simulink model "Assingment3_3K04_Part1"  (R2017b)
settings: Solver=FixedStepAuto  StartTime=0.0  StopTime=2  FixedStep=1e-3  RelTol=1e-3
undefined symbols (not defined in the file): A0, A1, D0, D1, D10, D11, D12, D13, D2, D3, D4, D5, D6, D7, D8, D9, PTA0, PTA1, PTA2, PTB2, PTB23, PTB3, PTB9, PTC16, PTC17, PTC2, PTC3, PTC4, PTD0, PTD1, PTD2, PTD3
libraries: frdmk64flib x25
settings Model: ExtModeTrigDuration=5  Creator=gagiche  LastModifiedBy=gagiche
settings DataIOCC: LimitDataPoints=on  SaveFormat=Array
settings OptimizationCC: PassReuseOutputArgsAs=Individual arguments  MaxStackSize=64
settings DebuggingCC: UnderspecifiedInitializationDetection=Classic  MergeDetectMultiDrivingBlocksExec=none  SolverPrmCheckMsg=warning  ParameterTunabilityLossMsg=error  StateNameClashWarn=warning  SFUnexpectedBacktrackingDiag=warning  SFNoUnconditionalDefaultTransitionDiag=warning  SFExecutionAtInitializationDiag=none
settings HardwareCC: ProdBitPerPointer=32  ProdBitPerSizeT=32  ProdBitPerPtrDiffT=32  ProdLargestAtomicInteger=Long  ProdLargestAtomicFloat=Double  ProdWordSize=32  ProdHWDeviceType=ARM Compatible->ARM Cortex
settings ModelReferenceCC: PropagateSignalLabelsOutOfModel=off
settings SFSimCC: MATLABDynamicMemAlloc=off
settings RTWCC: SystemTargetFile=ert.tlc  HardwareBoard=NXP FRDM-K64F  TemplateMakefile=ert_default_tmf  GenerateReport=on  Toolchain=GNU Tools for ARM Embedded Processors  IncludeHyperlinkInReport=on  LaunchReport=on  GenerateTraceInfo=on  GenerateTraceReport=on  GenerateTraceReportSl=on  GenerateTraceReportSf=on  GenerateTraceReportEml=on
settings CodeAppCC: ForceParamTrailComments=on  IgnoreCustomStorageClasses=off  OperatorAnnotations=on  SimulinkDataObjDesc=on  SFDataObjDesc=on  InsertBlockDesc=on
settings ConfigComp: CovMetricSettings=dw  CovHtmlReporting=on  CovSaveCumulativeToWorkspaceVar=on  CovSaveSingleToWorkspaceVar=on  CovExternalEMLEnable=off
settings SimscapeCC: SimscapeNormalizeSystem=off

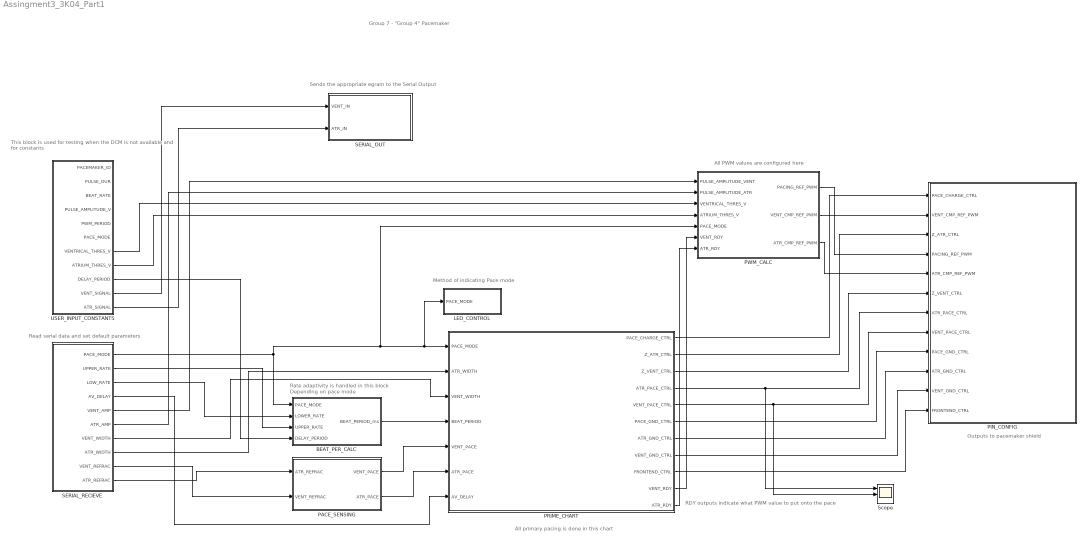
== system Assingment3_3K04_Part1 ==
  note: Group 7 - "Group 4" Pacemaker
  note: RDY outputs indicate what PWM value to put onto the pace
  note: Outputs to pacemaker shield
  note: All primary pacing is done in this chart
  note: Method of indicating Pace mode
  note: Rate adaptivity is handled in this block
      | Depending on pace mode
  note: Sends the appropriate egram to the Serial Output
  note: This block is used for testing when the DCM is not available
      | and for constants
  note: All PWM values are configured here
  note: Read serial data and set default parameters
  BEAT_PER_CALC : Subsystem
  LED_CONTROL : Subsystem
  PACE_SENSING : Subsystem
  "PIN_CONFIG " : Subsystem
  PRIME_CHART : Stateflow chart  TreatAsAtomicUnit=on
  PWM_CALC : Subsystem
  SERIAL_OUT : Subsystem
  SERIAL_RECIEVE : Subsystem
  Scope : Scope  NumInputPorts=3
  USER_INPUT_CONSTANTS : Subsystem
  wires:
  PRIME_CHART/1(PACE_CHARGE_CTRL) -> "PIN_CONFIG "/1(PACE_CHARGE_CTRL)
  PRIME_CHART/2(Z_ATR_CTRL) -> "PIN_CONFIG "/3(Z_ATR_CTRL)
  PRIME_CHART/4(ATR_PACE_CTRL) -> "PIN_CONFIG "/7(ATR_PACE_CTRL), Scope/1
  PRIME_CHART/3(Z_VENT_CTRL) -> "PIN_CONFIG "/6(Z_VENT_CTRL)
  PRIME_CHART/5(VENT_PACE_CTRL) -> Scope/2, "PIN_CONFIG "/8(VENT_PACE_CTRL)
  PRIME_CHART/6(PACE_GND_CTRL) -> "PIN_CONFIG "/9(PACE_GND_CTRL)
  PRIME_CHART/7(ATR_GND_CTRL) -> "PIN_CONFIG "/10(ATR_GND_CTRL)
  PRIME_CHART/8(VENT_GND_CTRL) -> "PIN_CONFIG "/11(VENT_GND_CTRL)
  PRIME_CHART/9(FRONTEND_CTRL) -> "PIN_CONFIG "/12(FRONTEND_CTRL)
  PACE_SENSING/1(VENT_PACE) -> PRIME_CHART/5(VENT_PACE)
  PACE_SENSING/2(ATR_PACE) -> PRIME_CHART/6(ATR_PACE)
  PWM_CALC/2(VENT_CMP_REF_PWM) -> "PIN_CONFIG "/2(VENT_CMP_REF_PWM)
  PWM_CALC/3(ATR_CMP_REF_PWM) -> "PIN_CONFIG "/5(ATR_CMP_REF_PWM)
  PWM_CALC/1(PACING_REF_PWM) -> "PIN_CONFIG "/4(PACING_REF_PWM)
  USER_INPUT_CONSTANTS/7(VENTRICAL_THRES_V) -> PWM_CALC/3(VENTRICAL_THRES_V)
  USER_INPUT_CONSTANTS/8(ATRIUM_THRES_V) -> PWM_CALC/4(ATRIUM_THRES_V)
  SERIAL_RECIEVE/1(PACE_MODE) -> PWM_CALC/5(PACE_MODE), LED_CONTROL/1(PACE_MODE), PRIME_CHART/1(PACE_MODE), BEAT_PER_CALC/1(PACE_MODE)
  SERIAL_RECIEVE/7(VENT_WIDTH) -> PRIME_CHART/3(VENT_WIDTH)
  SERIAL_RECIEVE/3(LOW_RATE) -> BEAT_PER_CALC/2(LOWER_RATE)
  SERIAL_RECIEVE/5(VENT_AMP) -> PWM_CALC/1("PULSE_AMPLITUDE_VENT ")
  SERIAL_RECIEVE/8(ATR_WIDTH) -> PRIME_CHART/2(ATR_WIDTH)
  SERIAL_RECIEVE/9(VENT_REFRAC) -> PACE_SENSING/2(VENT_REFRAC)
  SERIAL_RECIEVE/10(ATR_REFRAC) -> PACE_SENSING/1(ATR_REFRAC)
  SERIAL_RECIEVE/2(UPPER_RATE) -> BEAT_PER_CALC/3(UPPER_RATE)
  SERIAL_RECIEVE/6(ATR_AMP) -> PWM_CALC/2(PULSE_AMPLITUDE_ATR)
  BEAT_PER_CALC/1(BEAT_PERIOD_ms) -> PRIME_CHART/4(BEAT_PERIOD)
  USER_INPUT_CONSTANTS/9(DELAY_PERIOD) -> BEAT_PER_CALC/4(DELAY_PERIOD)
  SERIAL_RECIEVE/4(AV_DELAY) -> PRIME_CHART/7(AV_DELAY)
  PRIME_CHART/10(VENT_RDY) -> PWM_CALC/6(VENT_RDY)
  PRIME_CHART/11(ATR_RDY) -> PWM_CALC/7(ATR_RDY)
  USER_INPUT_CONSTANTS/10(VENT_SIGNAL) -> SERIAL_OUT/1(VENT_IN)
  USER_INPUT_CONSTANTS/11(ATR_SIGNAL) -> SERIAL_OUT/2(ATR_IN)

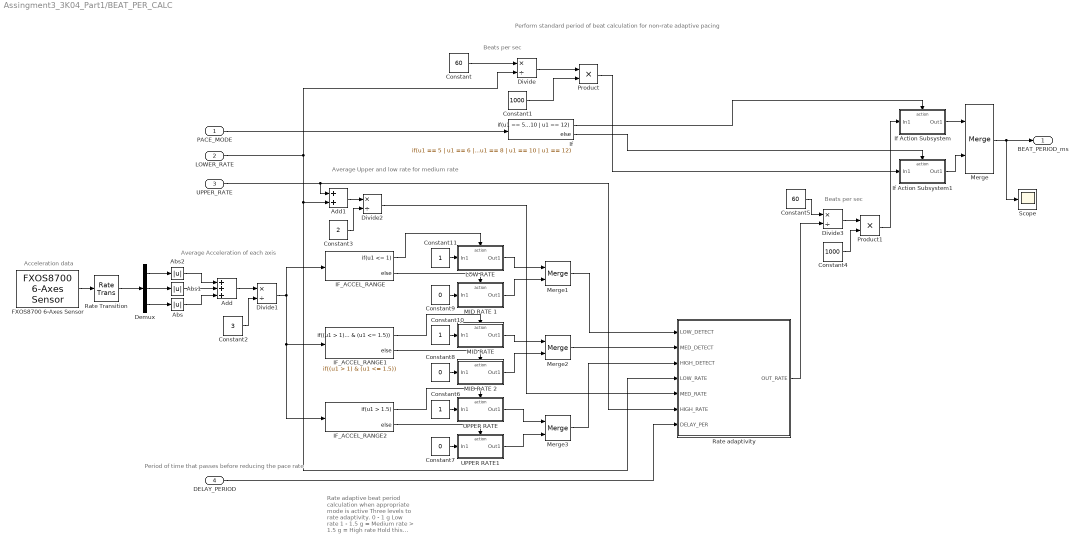
== system Assingment3_3K04_Part1/BEAT_PER_CALC ==
  note: Period of time that passes before reducing the pace rate
  note: Average Upper and low rate for medium rate
  note: Average Acceleration of each axis
  note: Acceleration data
  note: Rate adaptive beat period calculation when appropriate mode is active
      | Three levels to rate adaptivity.
      | 0 - 1 g Low rate
      | 1 - 1.5 g = Medium rate
      | > 1.5 g = High rate
      |
      | Hold this rate for delay_period mseconds
  note: Perform standard period of beat calculation for non-rate adaptive pacing
  note: Beats per sec
  note: Beats per sec
  PACE_MODE : Inport
  LOWER_RATE : Inport  Port=2
  UPPER_RATE : Inport  Port=3
  DELAY_PERIOD : Inport  Port=4
  Abs : Abs  RndMeth=Nearest
  Abs1 : Abs  RndMeth=Nearest
  Abs2 : Abs  RndMeth=Nearest
  Add : Sum  Inputs=3
  Add1 : Sum
  Constant : Constant  Value=60  OutDataTypeStr=double
  Constant1 : Constant  Value=1000  OutDataTypeStr=uint32
  Constant10 : Constant  OutDataTypeStr=double
  Constant11 : Constant  OutDataTypeStr=double
  Constant2 : Constant  Value=3  OutDataTypeStr=double
  Constant3 : Constant  Value=2  OutDataTypeStr=uint8
  Constant4 : Constant  Value=1000  OutDataTypeStr=uint32
  Constant5 : Constant  Value=60  OutDataTypeStr=double
  Constant6 : Constant  OutDataTypeStr=double
  Constant7 : Constant  Value=0  OutDataTypeStr=double
  Constant8 : Constant  Value=0  OutDataTypeStr=double
  Constant9 : Constant  Value=0  OutDataTypeStr=double
  Demux : Demux  Outputs=3
  Divide : Product  Inputs=*/  OutDataTypeStr=double
  Divide1 : Product  Inputs=*/
  Divide2 : Product  Inputs=*/  OutDataTypeStr=uint8
  Divide3 : Product  Inputs=*/  OutDataTypeStr=double
  FXOS8700 6-Axes Sensor : frdmk64flib/FXOS8700 6-Axes Sensor  Activesensor=Accelerometer only  ODR=12.5Hz  HybridODR=400Hz  Accelfullrange=-4g to +4g  SampleTime=0.1
      settings: SourceProductName=Simulink Coder Support Package for NXP FRDM-K64F Board
  IF_ACCEL_RANGE : If  IfExpression=u1 <= 1
  IF_ACCEL_RANGE1 : If  IfExpression=(u1 > 1) & (u1 <= 1.5)
  IF_ACCEL_RANGE2 : If  IfExpression=u1 > 1.5
  If : If  IfExpression=u1 == 5 | u1 == 6 | u1 == 7 | u1 == 8 | u1 == 10 | u1 == 12
  If Action Subsystem : Subsystem  TreatAsAtomicUnit=on
  If Action Subsystem1 : Subsystem  TreatAsAtomicUnit=on
  LOW RATE : Subsystem  TreatAsAtomicUnit=on
  MID RATE : Subsystem  TreatAsAtomicUnit=on
  MID RATE 1 : Subsystem  TreatAsAtomicUnit=on
  MID RATE 2 : Subsystem  TreatAsAtomicUnit=on
  Merge{,1..3} (4 alike) : Merge
  Product : Product  OutDataTypeStr=double
  Product1 : Product  OutDataTypeStr=double
  Rate Transition : RateTransition  OutPortSampleTime=0.001
  Rate adaptivity : Stateflow chart  TreatAsAtomicUnit=on
  Scope : Scope
  UPPER RATE : Subsystem  TreatAsAtomicUnit=on
  UPPER RATE1 : Subsystem  TreatAsAtomicUnit=on
  BEAT_PERIOD_ms : Outport  OutDataTypeStr=double
  wires:
  Divide/1 -> Product/1
  Constant1/1 -> Product/2
  LOWER_RATE/1 -> Rate adaptivity/4(LOW_RATE), Add1/2, Divide/2
  Constant/1 -> Divide/1
  If Action Subsystem/1(Out1) -> Merge/1
  If Action Subsystem1/1(Out1) -> Merge/2
  Merge/1 -> Scope/1, BEAT_PERIOD_ms/1
  PACE_MODE/1 -> If/1
  Demux/2 -> Abs1/1
  Demux/3 -> Abs/1
  Constant2/1 -> Divide1/2
  Demux/1 -> Abs2/1
  Abs2/1 -> Add/1
  Abs1/1 -> Add/2
  Abs/1 -> Add/3
  Add/1 -> Divide1/1
  Divide1/1 -> IF_ACCEL_RANGE2/1, IF_ACCEL_RANGE1/1, IF_ACCEL_RANGE/1
  Product/1 -> If Action Subsystem1/1(In1)
  If/2 -> If Action Subsystem1/Action
  If/1 -> If Action Subsystem/Action
  UPPER_RATE/1 -> Rate adaptivity/6(HIGH_RATE), Add1/1
  Constant3/1 -> Divide2/2
  Add1/1 -> Divide2/1
  Divide3/1 -> Product1/1
  Constant4/1 -> Product1/2
  Constant5/1 -> Divide3/1
  Product1/1 -> If Action Subsystem/1(In1)
  Divide2/1 -> Rate adaptivity/5(MED_RATE)
  IF_ACCEL_RANGE2/1 -> UPPER RATE/Action
  IF_ACCEL_RANGE2/2 -> UPPER RATE1/Action
  Constant6/1 -> UPPER RATE/1(In1)
  Constant7/1 -> UPPER RATE1/1(In1)
  IF_ACCEL_RANGE1/1 -> MID RATE/Action
  Constant8/1 -> MID RATE 2/1(In1)
  IF_ACCEL_RANGE1/2 -> MID RATE 2/Action
  IF_ACCEL_RANGE/1 -> LOW RATE/Action
  IF_ACCEL_RANGE/2 -> MID RATE 1/Action
  Constant9/1 -> MID RATE 1/1(In1)
  Constant10/1 -> MID RATE/1(In1)
  Constant11/1 -> LOW RATE/1(In1)
  LOW RATE/1(Out1) -> Merge1/1
  MID RATE 1/1(Out1) -> Merge1/2
  Merge1/1 -> Rate adaptivity/1(LOW_DETECT)
  Merge2/1 -> Rate adaptivity/2(MED_DETECT)
  MID RATE/1(Out1) -> Merge2/1
  MID RATE 2/1(Out1) -> Merge2/2
  UPPER RATE/1(Out1) -> Merge3/1
  UPPER RATE1/1(Out1) -> Merge3/2
  Merge3/1 -> Rate adaptivity/3(HIGH_DETECT)
  DELAY_PERIOD/1 -> Rate adaptivity/7(DELAY_PER)
  Rate adaptivity/1(OUT_RATE) -> Divide3/2
  FXOS8700 6-Axes Sensor/1 -> Rate Transition/1
  Rate Transition/1 -> Demux/1

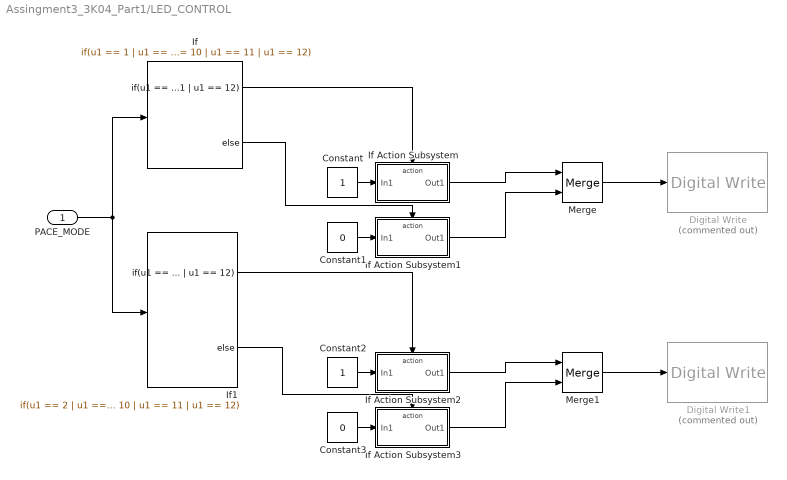
== system Assingment3_3K04_Part1/LED_CONTROL ==
  PACE_MODE : Inport
  Constant : Constant  OutDataTypeStr=boolean
  Constant1 : Constant  Value=0  OutDataTypeStr=boolean
  Constant2 : Constant  OutDataTypeStr=boolean
  Constant3 : Constant  Value=0  OutDataTypeStr=boolean
  Digital Write : frdmk64flib/Digital Write  Commented=on  Whichpin=GREEN_LED
      settings: SourceProductName=Simulink Coder Support Package for NXP FRDM-K64F Board
  Digital Write1 : frdmk64flib/Digital Write  Commented=on  Whichpin=RED_LED
      settings: SourceProductName=Simulink Coder Support Package for NXP FRDM-K64F Board
  If : If  IfExpression=u1 == 1 | u1 == 3 | u1 == 5 | u1 == 7 | u1 == 9 | u1 == 10 | u1 == 11 | u1 == 12
  If Action Subsystem : Subsystem  TreatAsAtomicUnit=on
  If Action Subsystem1 : Subsystem  TreatAsAtomicUnit=on
  If Action Subsystem2 : Subsystem  TreatAsAtomicUnit=on
  If Action Subsystem3 : Subsystem  TreatAsAtomicUnit=on
  If1 : If  IfExpression=u1 == 2 | u1 == 4 | u1 == 6 | u1 == 8 | u1 == 9 | u1 == 10 | u1 == 11 | u1 == 12
  Merge : Merge
  Merge1 : Merge
  wires:
  PACE_MODE/1 -> If1/1, If/1
  If/1 -> If Action Subsystem/Action
  If/2 -> If Action Subsystem1/Action
  Constant/1 -> If Action Subsystem/1(In1)
  Constant1/1 -> If Action Subsystem1/1(In1)
  Merge/1 -> Digital Write/1
  If Action Subsystem/1(Out1) -> Merge/1
  If Action Subsystem1/1(Out1) -> Merge/2
  Constant3/1 -> If Action Subsystem3/1(In1)
  If Action Subsystem3/1(Out1) -> Merge1/2
  If Action Subsystem2/1(Out1) -> Merge1/1
  Constant2/1 -> If Action Subsystem2/1(In1)
  Merge1/1 -> Digital Write1/1
  If1/2 -> If Action Subsystem3/Action
  If1/1 -> If Action Subsystem2/Action

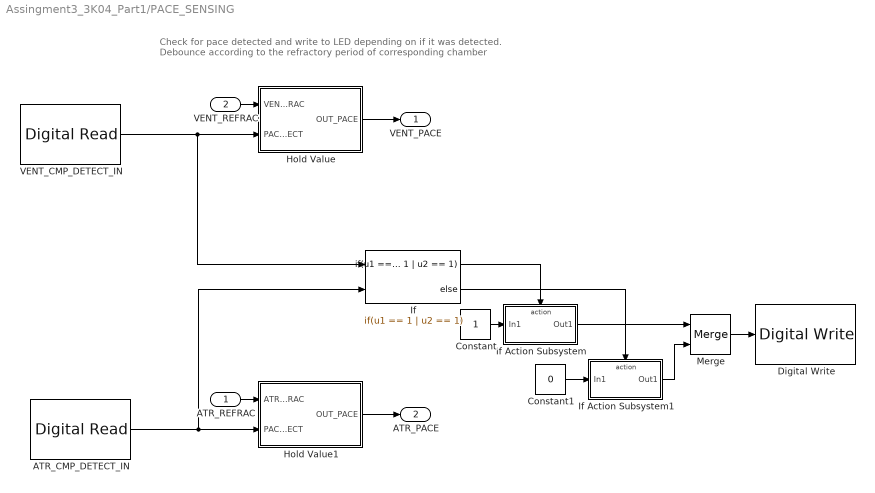
== system Assingment3_3K04_Part1/PACE_SENSING ==
  note: Check for pace detected and write to LED depending on if it was detected.
      | Debounce according to the refractory period of corresponding chamber
  ATR_REFRAC : Inport
  VENT_REFRAC : Inport  Port=2
  ATR_CMP_DETECT_IN : frdmk64flib/Digital Read  Whichpin=PTC16 (D0)  SampleTime=-1
      settings: SourceProductName=Simulink Coder Support Package for NXP FRDM-K64F Board
  Constant : Constant
  Constant1 : Constant  Value=0
  Digital Write : frdmk64flib/Digital Write  Whichpin=GREEN_LED
      settings: SourceProductName=Simulink Coder Support Package for NXP FRDM-K64F Board
  Hold Value : Stateflow chart  TreatAsAtomicUnit=on
  Hold Value1 : Stateflow chart  TreatAsAtomicUnit=on
  If : If  NumInputs=2  IfExpression=u1 == 1 | u2 == 1
  If Action Subsystem : Subsystem  TreatAsAtomicUnit=on
  If Action Subsystem1 : Subsystem  TreatAsAtomicUnit=on
  Merge : Merge
  VENT_CMP_DETECT_IN : frdmk64flib/Digital Read  Whichpin=PTC17 (D1)  SampleTime=-1
      settings: SourceProductName=Simulink Coder Support Package for NXP FRDM-K64F Board
  VENT_PACE : Outport  OutDataTypeStr=boolean
  ATR_PACE : Outport  Port=2  OutDataTypeStr=boolean
  wires:
  VENT_CMP_DETECT_IN/1 -> Hold Value/2(PACE_DETECT), If/1
  Merge/1 -> Digital Write/1
  If/1 -> If Action Subsystem/Action
  Constant/1 -> If Action Subsystem/1(In1)
  Constant1/1 -> If Action Subsystem1/1(In1)
  If/2 -> If Action Subsystem1/Action
  If Action Subsystem1/1(Out1) -> Merge/2
  If Action Subsystem/1(Out1) -> Merge/1
  ATR_CMP_DETECT_IN/1 -> If/2, Hold Value1/2(PACE_DETECT)
  VENT_REFRAC/1 -> Hold Value/1(VENT_REFRAC)
  Hold Value/1(OUT_PACE) -> VENT_PACE/1
  ATR_REFRAC/1 -> Hold Value1/1(ATR_REFRAC)
  Hold Value1/1(OUT_PACE) -> ATR_PACE/1

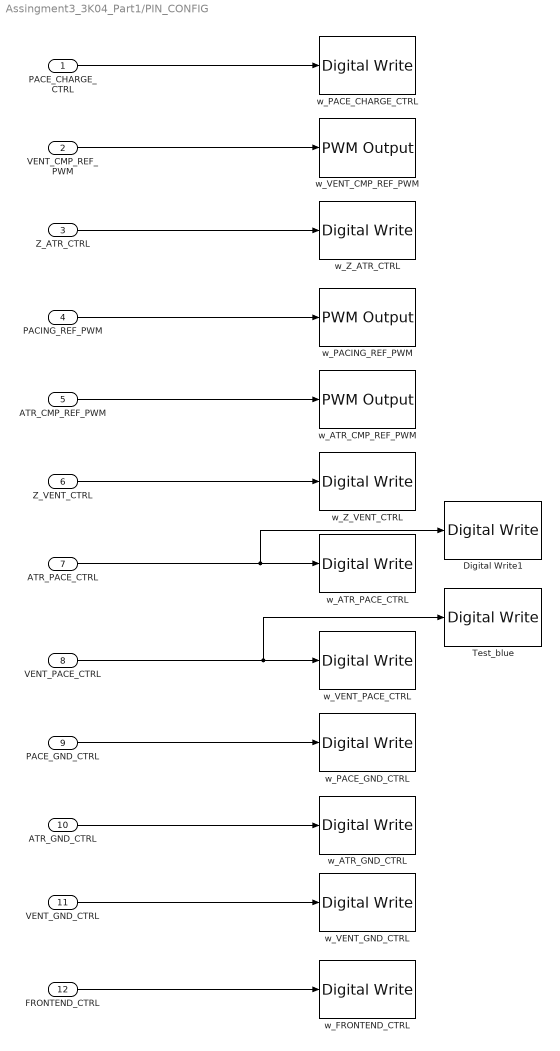
== system Assingment3_3K04_Part1/PIN_CONFIG  ==
  PACE_CHARGE_CTRL : Inport
  VENT_CMP_REF_PWM : Inport  Port=2
  Z_ATR_CTRL : Inport  Port=3
  PACING_REF_PWM : Inport  Port=4
  ATR_CMP_REF_PWM : Inport  Port=5
  Z_VENT_CTRL : Inport  Port=6
  ATR_PACE_CTRL : Inport  Port=7
  VENT_PACE_CTRL : Inport  Port=8
  PACE_GND_CTRL : Inport  Port=9
  ATR_GND_CTRL : Inport  Port=10
  VENT_GND_CTRL : Inport  Port=11
  FRONTEND_CTRL : Inport  Port=12
  Digital Write1 : frdmk64flib/Digital Write  Whichpin=RED_LED
      settings: SourceProductName=Simulink Coder Support Package for NXP FRDM-K64F Board
  Test_blue : frdmk64flib/Digital Write  Whichpin=BLUE_LED
      settings: SourceProductName=Simulink Coder Support Package for NXP FRDM-K64F Board
  w_ATR_CMP_REF_PWM : frdmk64flib/PWM Output  Whichpin=PTC2 (D6)  InitialFrequency=1000  InitialDutyCycle=0
      settings: SourceProductName=Simulink Coder Support Package for NXP FRDM-K64F Board
  w_ATR_GND_CTRL : frdmk64flib/Digital Write  Whichpin=PTD2 (D11)
      settings: SourceProductName=Simulink Coder Support Package for NXP FRDM-K64F Board
  w_ATR_PACE_CTRL : frdmk64flib/Digital Write  Whichpin=PTA0 (D8)
      settings: SourceProductName=Simulink Coder Support Package for NXP FRDM-K64F Board
  w_FRONTEND_CTRL : frdmk64flib/Digital Write  Whichpin=PTD1 (D13)
      settings: SourceProductName=Simulink Coder Support Package for NXP FRDM-K64F Board
  w_PACE_CHARGE_CTRL : frdmk64flib/Digital Write  Whichpin=PTB9 (D2)
      settings: SourceProductName=Simulink Coder Support Package for NXP FRDM-K64F Board
  w_PACE_GND_CTRL : frdmk64flib/Digital Write  Whichpin=PTD0 (D10)
      settings: SourceProductName=Simulink Coder Support Package for NXP FRDM-K64F Board
  w_PACING_REF_PWM : frdmk64flib/PWM Output  Whichpin=PTA2 (D5)  InitialFrequency=1000  InitialDutyCycle=0
      settings: SourceProductName=Simulink Coder Support Package for NXP FRDM-K64F Board
  w_VENT_CMP_REF_PWM : frdmk64flib/PWM Output  Whichpin=PTA1 (D3)  InitialFrequency=1000  InitialDutyCycle=0
      settings: SourceProductName=Simulink Coder Support Package for NXP FRDM-K64F Board
  w_VENT_GND_CTRL : frdmk64flib/Digital Write  Whichpin=PTD3 (D12)
      settings: SourceProductName=Simulink Coder Support Package for NXP FRDM-K64F Board
  w_VENT_PACE_CTRL : frdmk64flib/Digital Write  Whichpin=PTC4 (D9)
      settings: SourceProductName=Simulink Coder Support Package for NXP FRDM-K64F Board
  w_Z_ATR_CTRL : frdmk64flib/Digital Write  Whichpin=PTB23 (D4)
      settings: SourceProductName=Simulink Coder Support Package for NXP FRDM-K64F Board
  w_Z_VENT_CTRL : frdmk64flib/Digital Write  Whichpin=PTC3 (D7)
      settings: SourceProductName=Simulink Coder Support Package for NXP FRDM-K64F Board
  wires:
  PACE_CHARGE_CTRL/1 -> w_PACE_CHARGE_CTRL/1
  VENT_CMP_REF_PWM/1 -> w_VENT_CMP_REF_PWM/1
  Z_ATR_CTRL/1 -> w_Z_ATR_CTRL/1
  PACING_REF_PWM/1 -> w_PACING_REF_PWM/1
  ATR_CMP_REF_PWM/1 -> w_ATR_CMP_REF_PWM/1
  Z_VENT_CTRL/1 -> w_Z_VENT_CTRL/1
  ATR_PACE_CTRL/1 -> Digital Write1/1, w_ATR_PACE_CTRL/1
  VENT_PACE_CTRL/1 -> Test_blue/1, w_VENT_PACE_CTRL/1
  PACE_GND_CTRL/1 -> w_PACE_GND_CTRL/1
  ATR_GND_CTRL/1 -> w_ATR_GND_CTRL/1
  VENT_GND_CTRL/1 -> w_VENT_GND_CTRL/1
  FRONTEND_CTRL/1 -> w_FRONTEND_CTRL/1

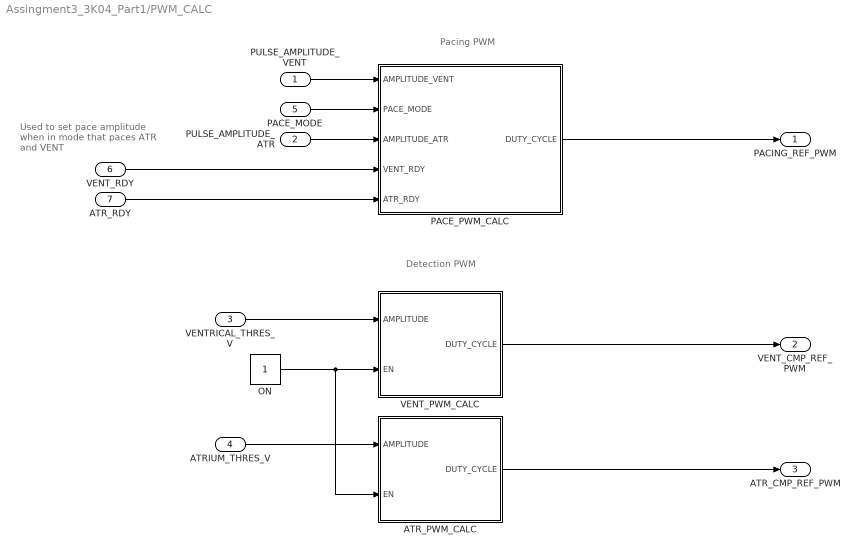
== system Assingment3_3K04_Part1/PWM_CALC ==
  note: Used to set pace amplitude
      | when in mode that paces ATR and VENT
  note: Pacing PWM
  note: Detection PWM
  "PULSE_AMPLITUDE_VENT " : Inport
  PULSE_AMPLITUDE_ATR : Inport  Port=2
  VENTRICAL_THRES_V : Inport  Port=3
  ATRIUM_THRES_V : Inport  Port=4
  PACE_MODE : Inport  Port=5
  VENT_RDY : Inport  Port=6
  ATR_RDY : Inport  Port=7
  ATR_PWM_CALC : Subsystem
  ON : Constant  OutDataTypeStr=boolean
  PACE_PWM_CALC : Subsystem
  VENT_PWM_CALC : Subsystem
  PACING_REF_PWM : Outport
  VENT_CMP_REF_PWM : Outport  Port=2
  ATR_CMP_REF_PWM : Outport  Port=3
  wires:
  ON/1 -> ATR_PWM_CALC/2(EN), VENT_PWM_CALC/2(EN)
  "PULSE_AMPLITUDE_VENT "/1 -> PACE_PWM_CALC/1(AMPLITUDE_VENT)
  VENTRICAL_THRES_V/1 -> VENT_PWM_CALC/1(AMPLITUDE)
  ATRIUM_THRES_V/1 -> ATR_PWM_CALC/1(AMPLITUDE)
  ATR_PWM_CALC/1(DUTY_CYCLE) -> ATR_CMP_REF_PWM/1
  VENT_PWM_CALC/1(DUTY_CYCLE) -> VENT_CMP_REF_PWM/1
  PACE_PWM_CALC/1(DUTY_CYCLE) -> PACING_REF_PWM/1
  PULSE_AMPLITUDE_ATR/1 -> PACE_PWM_CALC/3(AMPLITUDE_ATR)
  PACE_MODE/1 -> PACE_PWM_CALC/2(PACE_MODE)
  VENT_RDY/1 -> PACE_PWM_CALC/4(VENT_RDY)
  ATR_RDY/1 -> PACE_PWM_CALC/5(ATR_RDY)

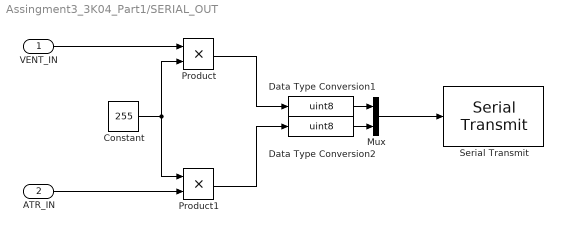
== system Assingment3_3K04_Part1/SERIAL_OUT ==
  VENT_IN : Inport
  ATR_IN : Inport  Port=2
  Constant : Constant  Value=255
  Data Type Conversion1 : DataTypeConversion  OutDataTypeStr=uint8
  Data Type Conversion2 : DataTypeConversion  OutDataTypeStr=uint8
  Mux : Mux  Inputs=2
  Product : Product
  Product1 : Product
  Serial Transmit : frdmk64flib/Serial Transmit  SCIModule=0  Baudrate=uint32(9600)  Parity=None  StopBits=1  HardwareFlowControl=None  ByteOrder=LittleEndian  BlockingMode=on  OutputStatus=off
      settings: SourceProductName=Simulink Coder Support Package for NXP FRDM-K64F Board
  wires:
  Constant/1 -> Product1/1, Product/2
  Product/1 -> Data Type Conversion1/1
  Product1/1 -> Data Type Conversion2/1
  Data Type Conversion1/1 -> Mux/1
  Data Type Conversion2/1 -> Mux/2
  Mux/1 -> Serial Transmit/1
  VENT_IN/1 -> Product/1
  ATR_IN/1 -> Product1/2

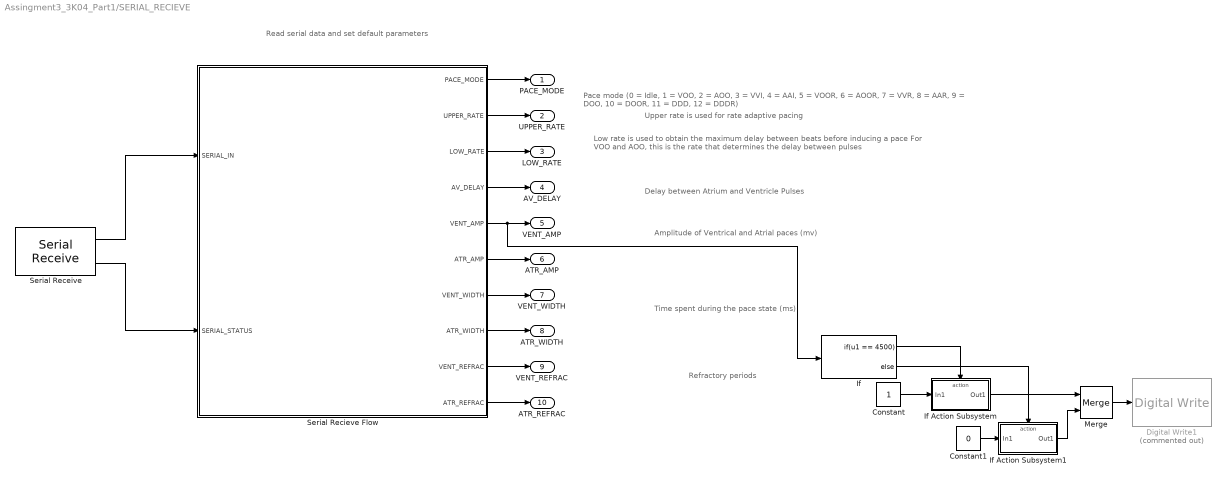
== system Assingment3_3K04_Part1/SERIAL_RECIEVE ==
  note: Read serial data and set default parameters
  note: Pace mode (0 = Idle, 1 = VOO, 2 = AOO, 3 = VVI, 4 = AAI, 5 = VOOR, 6 = AOOR, 7 = VVR, 8 = AAR, 9 = DOO, 10 = DOOR, 11 = DDD, 12 = DDDR)
  note: Amplitude of Ventrical and Atrial paces (mv)
  note: Delay between Atrium and Ventricle Pulses
  note: Refractory periods
  note: Upper rate is used for rate adaptive pacing
  note: Time spent during the pace state (ms)
  note: Low rate is used to obtain the maximum delay between beats before inducing a pace
      | For VOO and AOO, this is the rate that determines the delay between pulses
  Constant : Constant
  Constant1 : Constant  Value=0
  Digital Write1 : frdmk64flib/Digital Write  Commented=on  Whichpin=GREEN_LED
      settings: SourceProductName=Simulink Coder Support Package for NXP FRDM-K64F Board
  If : If  IfExpression=u1 == 4500
  If Action Subsystem : Subsystem  TreatAsAtomicUnit=on
  If Action Subsystem1 : Subsystem  TreatAsAtomicUnit=on
  Merge : Merge
  Serial Receive : frdmk64flib/Serial Receive  SCIModule=0  Baudrate=uint32(9600)  Parity=None  StopBits=1  HardwareFlowControl=None  ByteOrder=LittleEndian  DataType=uint8  DataLength=10  BlockingMode=off  OutputStatus=on  SampleTime=-1
      settings: SourceProductName=Simulink Coder Support Package for NXP FRDM-K64F Board
  Serial Recieve Flow : Stateflow chart  TreatAsAtomicUnit=on
  PACE_MODE : Outport  OutDataTypeStr=uint8
  UPPER_RATE : Outport  Port=2  OutDataTypeStr=uint8
  LOW_RATE : Outport  Port=3  OutDataTypeStr=uint8
  AV_DELAY : Outport  Port=4
  VENT_AMP : Outport  Port=5
  ATR_AMP : Outport  Port=6
  VENT_WIDTH : Outport  Port=7
  ATR_WIDTH : Outport  Port=8
  VENT_REFRAC : Outport  Port=9
  ATR_REFRAC : Outport  Port=10
  wires:
  Serial Recieve Flow/1(PACE_MODE) -> PACE_MODE/1
  Serial Recieve Flow/6(ATR_AMP) -> ATR_AMP/1
  Serial Recieve Flow/7(VENT_WIDTH) -> VENT_WIDTH/1
  Serial Recieve Flow/4(AV_DELAY) -> AV_DELAY/1
  Serial Recieve Flow/2(UPPER_RATE) -> UPPER_RATE/1
  Serial Recieve Flow/9(VENT_REFRAC) -> VENT_REFRAC/1
  Serial Recieve Flow/5(VENT_AMP) -> If/1, VENT_AMP/1
  Serial Recieve Flow/10(ATR_REFRAC) -> ATR_REFRAC/1
  Serial Recieve Flow/8(ATR_WIDTH) -> ATR_WIDTH/1
  Serial Recieve Flow/3(LOW_RATE) -> LOW_RATE/1
  If Action Subsystem1/1(Out1) -> Merge/2
  If/2 -> If Action Subsystem1/Action
  Constant/1 -> If Action Subsystem/1(In1)
  If/1 -> If Action Subsystem/Action
  Merge/1 -> Digital Write1/1
  Constant1/1 -> If Action Subsystem1/1(In1)
  If Action Subsystem/1(Out1) -> Merge/1
  Serial Receive/1 -> Serial Recieve Flow/1(SERIAL_IN)
  Serial Receive/2 -> Serial Recieve Flow/2(SERIAL_STATUS)

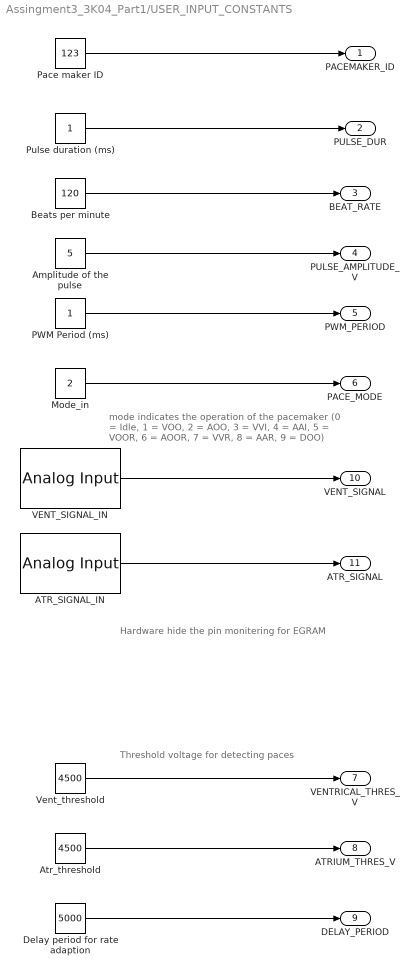
== system Assingment3_3K04_Part1/USER_INPUT_CONSTANTS ==
  note: Hardware hide the pin monitering for EGRAM
  note: Threshold voltage for detecting paces
  note: mode indicates the operation of the pacemaker
      | (0 = Idle, 1 = VOO, 2 = AOO, 3 = VVI, 4 = AAI, 5 = VOOR, 6 = AOOR, 7 = VVR, 8 = AAR, 9 = DOO)
  ATR_SIGNAL_IN : frdmk64flib/Analog Input  Whichpin=PTB2 (A0)  SampleTime=-1
      settings: SourceProductName=Simulink Coder Support Package for NXP FRDM-K64F Board
  Amplitude of the pulse : Constant  Value=5
  Atr_threshold : Constant  Value=4500  OutDataTypeStr=double
  Beats per minute : Constant  Value=120
  Delay period for rate adaption : Constant  Value=5000  OutDataTypeStr=double
  Mode_in : Constant  Value=2  OutDataTypeStr=uint16
  PWM Period (ms) : Constant  OutDataTypeStr=uint16
  Pace maker ID : Constant  Value=123  OutDataTypeStr=double
  Pulse duration (ms) : Constant  OutDataTypeStr=double
  VENT_SIGNAL_IN : frdmk64flib/Analog Input  Whichpin=PTB3 (A1)  SampleTime=-1
      settings: SourceProductName=Simulink Coder Support Package for NXP FRDM-K64F Board
  Vent_threshold : Constant  Value=4500  OutDataTypeStr=double
  PACEMAKER_ID : Outport  OutDataTypeStr=double
  "PULSE_DUR " : Outport  Port=2  OutDataTypeStr=double
  "BEAT_RATE " : Outport  Port=3
  "PULSE_AMPLITUDE_V " : Outport  Port=4
  PWM_PERIOD : Outport  Port=5
  PACE_MODE : Outport  Port=6
  VENTRICAL_THRES_V : Outport  Port=7
  ATRIUM_THRES_V : Outport  Port=8
  DELAY_PERIOD : Outport  Port=9
  VENT_SIGNAL : Outport  Port=10
  ATR_SIGNAL : Outport  Port=11
  wires:
  Pulse duration (ms)/1 -> "PULSE_DUR "/1
  Beats per minute/1 -> "BEAT_RATE "/1
  Amplitude of the pulse/1 -> "PULSE_AMPLITUDE_V "/1
  PWM Period (ms)/1 -> PWM_PERIOD/1
  Mode_in/1 -> PACE_MODE/1
  Vent_threshold/1 -> VENTRICAL_THRES_V/1
  Atr_threshold/1 -> ATRIUM_THRES_V/1
  Pace maker ID/1 -> PACEMAKER_ID/1
  Delay period for rate adaption/1 -> DELAY_PERIOD/1
  VENT_SIGNAL_IN/1 -> VENT_SIGNAL/1
  ATR_SIGNAL_IN/1 -> ATR_SIGNAL/1

== system Assingment3_3K04_Part1/BEAT_PER_CALC/If Action Subsystem ==
  In1 : Inport
  Action Port : ActionPort  ActionType=then
  Out1 : Outport
  wires:
  In1/1 -> Out1/1

== system Assingment3_3K04_Part1/BEAT_PER_CALC/If Action Subsystem1 ==
  In1 : Inport
  Action Port : ActionPort  ActionType=else
  Out1 : Outport
  wires:
  In1/1 -> Out1/1

== system Assingment3_3K04_Part1/BEAT_PER_CALC/LOW RATE ==
  In1 : Inport
  Action Port : ActionPort  ActionType=then
  Out1 : Outport
  wires:
  In1/1 -> Out1/1

== system Assingment3_3K04_Part1/BEAT_PER_CALC/MID RATE ==
  In1 : Inport
  Action Port : ActionPort  ActionType=then
  Out1 : Outport
  wires:
  In1/1 -> Out1/1

== system Assingment3_3K04_Part1/BEAT_PER_CALC/MID RATE 1 ==
  In1 : Inport
  Action Port : ActionPort  ActionType=else
  Out1 : Outport
  wires:
  In1/1 -> Out1/1

== system Assingment3_3K04_Part1/BEAT_PER_CALC/MID RATE 2 ==
  In1 : Inport
  Action Port : ActionPort  ActionType=else
  Out1 : Outport
  wires:
  In1/1 -> Out1/1

== system Assingment3_3K04_Part1/BEAT_PER_CALC/UPPER RATE ==
  In1 : Inport
  Action Port : ActionPort  ActionType=then
  Out1 : Outport
  wires:
  In1/1 -> Out1/1

== system Assingment3_3K04_Part1/BEAT_PER_CALC/UPPER RATE1 ==
  In1 : Inport
  Action Port : ActionPort  ActionType=else
  Out1 : Outport
  wires:
  In1/1 -> Out1/1

== system Assingment3_3K04_Part1/LED_CONTROL/If Action Subsystem ==
  In1 : Inport
  Action Port : ActionPort  ActionType=then
  Out1 : Outport
  wires:
  In1/1 -> Out1/1

== system Assingment3_3K04_Part1/LED_CONTROL/If Action Subsystem1 ==
  In1 : Inport
  Action Port : ActionPort  ActionType=else
  Out1 : Outport
  wires:
  In1/1 -> Out1/1

== system Assingment3_3K04_Part1/LED_CONTROL/If Action Subsystem2 ==
  In1 : Inport
  Action Port : ActionPort  ActionType=then
  Out1 : Outport
  wires:
  In1/1 -> Out1/1

== system Assingment3_3K04_Part1/LED_CONTROL/If Action Subsystem3 ==
  In1 : Inport
  Action Port : ActionPort  ActionType=else
  Out1 : Outport
  wires:
  In1/1 -> Out1/1

== system Assingment3_3K04_Part1/PACE_SENSING/If Action Subsystem ==
  In1 : Inport
  Action Port : ActionPort  ActionType=then
  Out1 : Outport
  wires:
  In1/1 -> Out1/1

== system Assingment3_3K04_Part1/PACE_SENSING/If Action Subsystem1 ==
  In1 : Inport
  Action Port : ActionPort  ActionType=else
  Out1 : Outport
  wires:
  In1/1 -> Out1/1

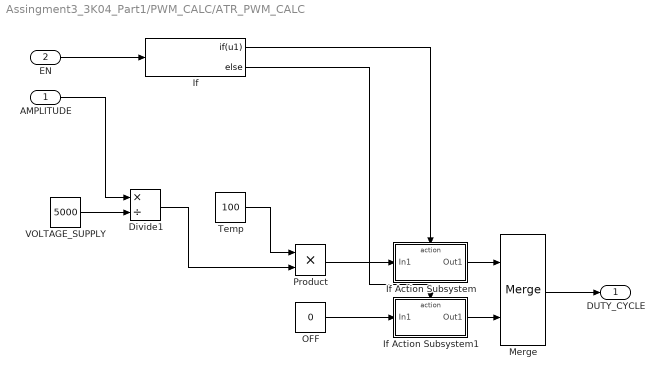
== system Assingment3_3K04_Part1/PWM_CALC/ATR_PWM_CALC ==
  AMPLITUDE : Inport  OutDataTypeStr=double
  EN : Inport  Port=2  OutDataTypeStr=boolean
  Divide1 : Product  Inputs=*/  OutDataTypeStr=double
  If : If  IfExpression=u1
  If Action Subsystem : Subsystem  TreatAsAtomicUnit=on
  If Action Subsystem1 : Subsystem  TreatAsAtomicUnit=on
  Merge : Merge
  OFF : Constant  Value=0  OutDataTypeStr=uint32
  Product : Product  OutDataTypeStr=uint32
  "Temp " : Constant  Value=100  OutDataTypeStr=double
  "VOLTAGE_SUPPLY " : Constant  Value=5000  OutDataTypeStr=double
  DUTY_CYCLE : Outport  OutDataTypeStr=uint32  LockScale=on
  wires:
  "VOLTAGE_SUPPLY "/1 -> Divide1/2
  "Temp "/1 -> Product/1
  EN/1 -> If/1
  Merge/1 -> DUTY_CYCLE/1
  If Action Subsystem/1(Out1) -> Merge/1
  If Action Subsystem1/1(Out1) -> Merge/2
  Product/1 -> If Action Subsystem/1(In1)
  If/1 -> If Action Subsystem/Action
  If/2 -> If Action Subsystem1/Action
  OFF/1 -> If Action Subsystem1/1(In1)
  AMPLITUDE/1 -> Divide1/1
  Divide1/1 -> Product/2

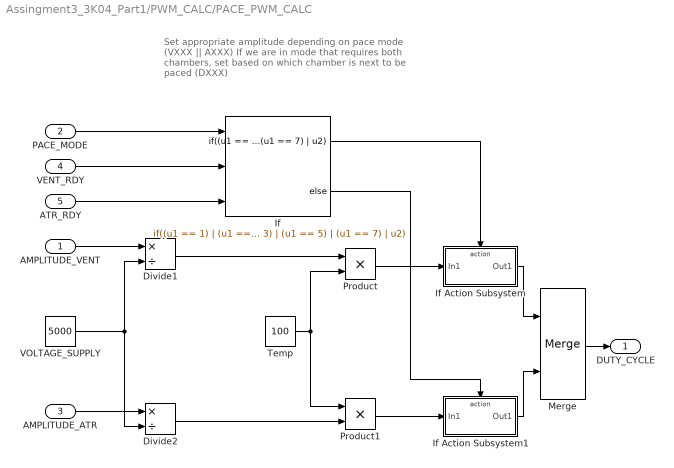
== system Assingment3_3K04_Part1/PWM_CALC/PACE_PWM_CALC ==
  note: Set appropriate amplitude depending on pace mode
      | (VXXX || AXXX)
      | If we are in mode that requires both chambers, set
      | based on which chamber is next to be paced
      | (DXXX)
  AMPLITUDE_VENT : Inport
  PACE_MODE : Inport  Port=2  OutDataTypeStr=uint8
  AMPLITUDE_ATR : Inport  Port=3  OutDataTypeStr=double
  VENT_RDY : Inport  Port=4
  ATR_RDY : Inport  Port=5
  Divide1 : Product  Inputs=*/  OutDataTypeStr=double
  Divide2 : Product  Inputs=*/  OutDataTypeStr=double
  If : If  NumInputs=3  IfExpression=(u1 == 1) | (u1 == 3) | (u1 == 5) | (u1 == 7) | u2
  If Action Subsystem : Subsystem  TreatAsAtomicUnit=on
  If Action Subsystem1 : Subsystem  TreatAsAtomicUnit=on
  Merge : Merge
  Product : Product  OutDataTypeStr=uint32
  Product1 : Product  OutDataTypeStr=uint32
  "Temp " : Constant  Value=100  OutDataTypeStr=double
  "VOLTAGE_SUPPLY " : Constant  Value=5000  OutDataTypeStr=double
  DUTY_CYCLE : Outport  OutDataTypeStr=uint32  LockScale=on
  wires:
  "VOLTAGE_SUPPLY "/1 -> Divide1/2, Divide2/2
  "Temp "/1 -> Product1/1, Product/2
  PACE_MODE/1 -> If/1
  If Action Subsystem/1(Out1) -> Merge/1
  If Action Subsystem1/1(Out1) -> Merge/2
  Product/1 -> If Action Subsystem/1(In1)
  If/1 -> If Action Subsystem/Action
  If/2 -> If Action Subsystem1/Action
  AMPLITUDE_VENT/1 -> Divide1/1
  Divide2/1 -> Product1/2
  AMPLITUDE_ATR/1 -> Divide2/1
  Product1/1 -> If Action Subsystem1/1(In1)
  Divide1/1 -> Product/1
  Merge/1 -> DUTY_CYCLE/1
  VENT_RDY/1 -> If/2
  ATR_RDY/1 -> If/3

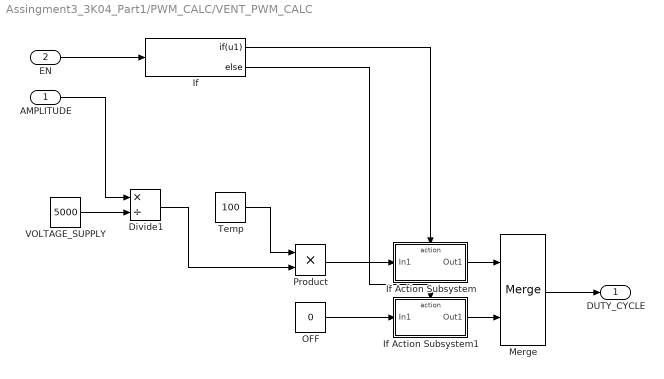
== system Assingment3_3K04_Part1/PWM_CALC/VENT_PWM_CALC ==
  AMPLITUDE : Inport  OutDataTypeStr=double
  EN : Inport  Port=2  OutDataTypeStr=boolean
  Divide1 : Product  Inputs=*/  OutDataTypeStr=double
  If : If  IfExpression=u1
  If Action Subsystem : Subsystem  TreatAsAtomicUnit=on
  If Action Subsystem1 : Subsystem  TreatAsAtomicUnit=on
  Merge : Merge
  OFF : Constant  Value=0  OutDataTypeStr=uint32
  Product : Product  OutDataTypeStr=uint32
  "Temp " : Constant  Value=100  OutDataTypeStr=double
  "VOLTAGE_SUPPLY " : Constant  Value=5000  OutDataTypeStr=double
  DUTY_CYCLE : Outport  OutDataTypeStr=uint32  LockScale=on
  wires:
  "VOLTAGE_SUPPLY "/1 -> Divide1/2
  "Temp "/1 -> Product/1
  EN/1 -> If/1
  Merge/1 -> DUTY_CYCLE/1
  If Action Subsystem/1(Out1) -> Merge/1
  If Action Subsystem1/1(Out1) -> Merge/2
  Product/1 -> If Action Subsystem/1(In1)
  If/1 -> If Action Subsystem/Action
  If/2 -> If Action Subsystem1/Action
  OFF/1 -> If Action Subsystem1/1(In1)
  AMPLITUDE/1 -> Divide1/1
  Divide1/1 -> Product/2

== system Assingment3_3K04_Part1/SERIAL_RECIEVE/If Action Subsystem ==
  In1 : Inport
  Action Port : ActionPort  ActionType=then
  Out1 : Outport
  wires:
  In1/1 -> Out1/1

== system Assingment3_3K04_Part1/SERIAL_RECIEVE/If Action Subsystem1 ==
  In1 : Inport
  Action Port : ActionPort  ActionType=else
  Out1 : Outport
  wires:
  In1/1 -> Out1/1

== system Assingment3_3K04_Part1/PWM_CALC/ATR_PWM_CALC/If Action Subsystem ==
  In1 : Inport
  Action Port : ActionPort  ActionType=then
  Out1 : Outport
  wires:
  In1/1 -> Out1/1

== system Assingment3_3K04_Part1/PWM_CALC/ATR_PWM_CALC/If Action Subsystem1 ==
  In1 : Inport
  Action Port : ActionPort  ActionType=else
  Out1 : Outport
  wires:
  In1/1 -> Out1/1

== system Assingment3_3K04_Part1/PWM_CALC/PACE_PWM_CALC/If Action Subsystem ==
  In1 : Inport
  Action Port : ActionPort  ActionType=then
  Out1 : Outport
  wires:
  In1/1 -> Out1/1

== system Assingment3_3K04_Part1/PWM_CALC/PACE_PWM_CALC/If Action Subsystem1 ==
  In1 : Inport
  Action Port : ActionPort  ActionType=else
  Out1 : Outport
  wires:
  In1/1 -> Out1/1

== system Assingment3_3K04_Part1/PWM_CALC/VENT_PWM_CALC/If Action Subsystem ==
  In1 : Inport
  Action Port : ActionPort  ActionType=then
  Out1 : Outport
  wires:
  In1/1 -> Out1/1

== system Assingment3_3K04_Part1/PWM_CALC/VENT_PWM_CALC/If Action Subsystem1 ==
  In1 : Inport
  Action Port : ActionPort  ActionType=else
  Out1 : Outport
  wires:
  In1/1 -> Out1/1

== stateflow chart Assingment3_3K04_Part1/BEAT_PER_CALC/Rate adaptivity ==
  settings: sampleTime=0.001
  note: Based on the detected acceleration, jump to the appropriate rate response
  state LOW_RATE
    entry:
    OUT_RATE = LOW_RATE;
  state MED_RATE
    entry:
    OUT_RATE = MED_RATE;
  note: Reduce the rate after a period of no accerlation corresponding to the rate
  state HIGH_RATE
    entry:
    OUT_RATE = HIGH_RATE;
  (default) -> LOW_RATE
  LOW_RATE -> LOW_RATE [order 3] : [after(200,msec)]
  MED_RATE -> LOW_RATE [order 2] : [after(DELAY_PER, msec)]
  LOW_RATE -> HIGH_RATE [order 1] : [HIGH_DETECT == 1]
  LOW_RATE -> MED_RATE [order 2] : [MED_DETECT == 1]
  MED_RATE -> MED_RATE [order 3] : [MED_DETECT == 1]
  HIGH_RATE -> MED_RATE [order 1] : [after(DELAY_PER, msec)]
  MED_RATE -> HIGH_RATE [order 1] : [HIGH_DETECT == 1]
  HIGH_RATE -> HIGH_RATE [order 2] : [HIGH_DETECT == 1]
  data: LOW_DETECT input; OUT_RATE output; MED_DETECT input; HIGH_DETECT input; LOW_RATE input; MED_RATE input; HIGH_RATE input; DELAY_PER input

== stateflow chart Assingment3_3K04_Part1/SERIAL_RECIEVE/Serial Recieve Flow ==
  settings: sampleTime=0.001  executeAtInitialization=1
  state DEFAULT
    entry:
    PACE_MODE = 1; %VVO
    UPPER_RATE = 160;
    LOW_RATE = 60;
    AV_DELAY = 300;
    VENT_AMP = 4500;
    ATR_AMP = 4500;
    VENT_WIDTH = 2;
    ATR_WIDTH = 2;
    VENT_REFRAC = 300;
    ATR_REFRAC = 300;
  note: Set default start-up values and then wait for updates via serial
  state WAIT_SERIAL
    %Wait for zero on status
    entry:
  state SERIAL_RECIEVE
    entry:
    PACE_MODE = SERIAL_IN(1);
    UPPER_RATE = SERIAL_IN(2);
    LOW_RATE = SERIAL_IN(3);
    AV_DELAY = double(SERIAL_IN(4))*10;
    VENT_AMP = double(SERIAL_IN(5))*100;
    ATR_AMP = double(SERIAL_IN(6))*100;
    VENT_WIDTH = double(SERIAL_IN(7));
    ATR_WIDTH = double(SERIAL_IN(8));
    VENT_REFRAC = double(SERIAL_IN(9))*10;
    ATR_REFRAC = double(SERIAL_IN(10))*10;
  note: New Serial Data to read
  (default) -> DEFAULT
  DEFAULT -> WAIT_SERIAL
  SERIAL_RECIEVE -> WAIT_SERIAL : [SERIAL_STATUS ~= 0]
  WAIT_SERIAL -> SERIAL_RECIEVE : [SERIAL_STATUS == 0]
  data: PACE_MODE output uint8; UPPER_RATE output uint8; LOW_RATE output uint8; SERIAL_IN input uint8; SERIAL_STATUS input uint8; AV_DELAY output double; VENT_AMP output double; ATR_AMP output double; VENT_WIDTH output double; ATR_WIDTH output double; VENT_REFRAC output double; ATR_REFRAC output double

== stateflow chart Assingment3_3K04_Part1/PRIME_CHART ==
  settings: sampleTime=0.001
  note: AOO/ AOOR mode
  note: DOOR and DOO
      |
      | Charge Atrium, discharge atrium, charge vent, wait av_delay, discharge vent, repeat
  state AOO_CHARGE
    entry:
    PACE_GND_CTRL = 1;
    ATR_PACE_CTRL = 0;
    Z_ATR_CTRL = 0;
    Z_VENT_CTRL = 0;
    VENT_PACE_CTRL = 0;
    VENT_GND_CTRL = 0;
    ATR_GND_CTRL = 1;
    FRONTEND_CTRL = 1;
    PACE_CHARGE_CTRL = 1;
  state AOO_DISCHARGE
    entry:
    PACE_CHARGE_CTRL = 0;
    PACE_GND_CTRL = 1;
    VENT_PACE_CTRL = 0;
    VENT_GND_CTRL = 0;
    Z_ATR_CTRL = 0;
    Z_VENT_CTRL = 0;
    ATR_GND_CTRL = 0;
    ATR_PACE_CTRL = 1;
    FRONTEND_CTRL = 1;
  state DOO_CHARGE_ATR
    entry:
    PACE_CHARGE_CTRL = 1;
    PACE_GND_CTRL = 1;
    VENT_PACE_CTRL = 0;
    Z_ATR_CTRL = 0;
    Z_VENT_CTRL = 0;
    ATR_PACE_CTRL = 0;
    ATR_GND_CTRL = 0;
    VENT_GND_CTRL = 1;
    FRONTEND_CTRL = 1;
    ATR_RDY = 1;
    VENT_RDY = 0;
  state DOO_DISCHARGE_ATR
    entry:
    PACE_CHARGE_CTRL = 0;
    PACE_GND_CTRL = 1;
    ATR_PACE_CTRL = 1;
    ATR_GND_CTRL = 0;
    Z_ATR_CTRL = 0;
    Z_VENT_CTRL = 0;
    VENT_GND_CTRL = 0;
    VENT_PACE_CTRL = 0;
    FRONTEND_CTRL = 1;
  note: VOO / VOOR Mode
  state VOO_CHARGE
    entry:
    PACE_GND_CTRL = 1;
    VENT_PACE_CTRL = 0;
    Z_ATR_CTRL = 0;
    Z_VENT_CTRL = 0;
    ATR_PACE_CTRL = 0;
    ATR_GND_CTRL = 0;
    VENT_GND_CTRL = 1;
    FRONTEND_CTRL = 1;
    PACE_CHARGE_CTRL = 1;
  state VOO_DISCHARGE
    entry:
    PACE_CHARGE_CTRL = 0;
    PACE_GND_CTRL = 1;
    ATR_PACE_CTRL = 0;
    ATR_GND_CTRL = 0;
    Z_ATR_CTRL = 0;
    Z_VENT_CTRL = 0;
    VENT_GND_CTRL = 0;
    VENT_PACE_CTRL = 1;
    FRONTEND_CTRL = 1;
  state DOO_CHARGE_VENT
    entry:
    PACE_CHARGE_CTRL = 1;
    PACE_GND_CTRL = 1;
    VENT_PACE_CTRL = 0;
    Z_ATR_CTRL = 0;
    Z_VENT_CTRL = 0;
    ATR_PACE_CTRL = 0;
    ATR_GND_CTRL = 1;
    VENT_GND_CTRL = 0;
    FRONTEND_CTRL = 1;
    ATR_RDY = 0;
    VENT_RDY = 1;
  state DOO_DISCHARGE_VENT
    entry:
    PACE_CHARGE_CTRL = 0;
    PACE_GND_CTRL = 1;
    ATR_PACE_CTRL = 0;
    ATR_GND_CTRL = 0;
    Z_ATR_CTRL = 0;
    Z_VENT_CTRL = 0;
    VENT_GND_CTRL = 0;
    VENT_PACE_CTRL = 1;
    FRONTEND_CTRL = 1;
  note: Remain here for a short period before change of mode
  state IDLE
    %All pace modes return here if there
    % is a change of mode
    entry:
    VENT_RDY = 0;
    ATR_RDY = 0;
  state VVI_CHARGE
    entry:
    PACE_GND_CTRL = 1;
    VENT_PACE_CTRL = 0;
    Z_ATR_CTRL = 0;
    Z_VENT_CTRL = 0;
    ATR_PACE_CTRL = 0;
    ATR_GND_CTRL = 0;
    VENT_GND_CTRL = 1;
    FRONTEND_CTRL = 1;
    PACE_CHARGE_CTRL = 1;
  state VVI_DISCHARGE
    entry:
    PACE_CHARGE_CTRL = 0;
    PACE_GND_CTRL = 1;
    ATR_PACE_CTRL = 0;
    ATR_GND_CTRL = 0;
    Z_ATR_CTRL = 0;
    Z_VENT_CTRL = 0;
    VENT_GND_CTRL = 0;
    VENT_PACE_CTRL = 1;
    FRONTEND_CTRL = 1;
  note: VVI / VVIR Mode
  note: DDDR and DDD
      |
      | Charge Atrium, discharge atrium, charge vent, wait av_delay, discharge vent, repeat
      | Don't pace if pace sensed
  note: If sense a pace, reset timers
  state AAI_CHARGE
    entry:
    PACE_GND_CTRL = 1;
    VENT_PACE_CTRL = 0;
    Z_ATR_CTRL = 0;
    Z_VENT_CTRL = 0;
    ATR_PACE_CTRL = 0;
    ATR_GND_CTRL = 1;
    VENT_GND_CTRL = 0;
    FRONTEND_CTRL = 1;
    PACE_CHARGE_CTRL = 1;
  note: AAI / AAIR MODE
  state DDD_CHARGE_ATR
    entry:
    PACE_CHARGE_CTRL = 1;
    PACE_GND_CTRL = 1;
    VENT_PACE_CTRL = 0;
    Z_ATR_CTRL = 0;
    Z_VENT_CTRL = 0;
    ATR_PACE_CTRL = 0;
    ATR_GND_CTRL = 0;
    VENT_GND_CTRL = 1;
    FRONTEND_CTRL = 1;
    ATR_RDY = 1;
    VENT_RDY = 0;
  state DDD_DISCHARGE_ATR
    entry:
    PACE_CHARGE_CTRL = 0;
    PACE_GND_CTRL = 1;
    ATR_PACE_CTRL = 1;
    ATR_GND_CTRL = 0;
    Z_ATR_CTRL = 0;
    Z_VENT_CTRL = 0;
    VENT_GND_CTRL = 0;
    VENT_PACE_CTRL = 0;
    FRONTEND_CTRL = 1;
  state AAI_DISCHARGE
    entry:
    PACE_CHARGE_CTRL = 0;
    PACE_GND_CTRL = 1;
    ATR_PACE_CTRL = 1;
    ATR_GND_CTRL = 0;
    Z_ATR_CTRL = 0;
    Z_VENT_CTRL = 0;
    VENT_GND_CTRL = 0;
    VENT_PACE_CTRL = 0;
    FRONTEND_CTRL = 1;
  note: If we sense a ATR pace dont pace ATR
  note: If we sense a VENT pace dont pace VENT
  note: If sense a pace, reset timers
  state DDD_CHARGE_VENT
    entry:
    PACE_CHARGE_CTRL = 1;
    PACE_GND_CTRL = 1;
    VENT_PACE_CTRL = 0;
    Z_ATR_CTRL = 0;
    Z_VENT_CTRL = 0;
    ATR_PACE_CTRL = 0;
    ATR_GND_CTRL = 1;
    VENT_GND_CTRL = 0;
    FRONTEND_CTRL = 1;
    ATR_RDY = 0;
    VENT_RDY = 1;
  state DDD_DISCHARGE_VENT
    entry:
    PACE_CHARGE_CTRL = 0;
    PACE_GND_CTRL = 1;
    ATR_PACE_CTRL = 0;
    ATR_GND_CTRL = 0;
    Z_ATR_CTRL = 0;
    Z_VENT_CTRL = 0;
    VENT_GND_CTRL = 0;
    VENT_PACE_CTRL = 1;
    FRONTEND_CTRL = 1;
  AOO_CHARGE -> IDLE [order 2] : [(PACE_MODE ~= 2) && (PACE_MODE ~= 6) ]
  IDLE -> AOO_CHARGE [order 2] : [(PACE_MODE == 2) || (PACE_MODE == 6)]
  AOO_CHARGE -> AOO_DISCHARGE [order 1] : after(BEAT_PERIOD - ATR_WIDTH, msec)
  IDLE -> DOO_CHARGE_ATR [order 7] : [(PACE_MODE == 9) || (PACE_MODE == 10)]
  AOO_DISCHARGE -> AOO_CHARGE : after(ATR_WIDTH, msec)
  DOO_CHARGE_ATR -> IDLE [order 1] : [(PACE_MODE ~= 9) && (PACE_MODE ~= 10)]
  DOO_CHARGE_ATR -> DOO_DISCHARGE_ATR [order 2] : [after(BEAT_PERIOD - AV_DELAY - VENT_WIDTH - ATR_WIDTH, msec)]
  VOO_CHARGE -> IDLE [order 2] : [(PACE_MODE ~= 1) && (PACE_MODE ~= 5)]
  DOO_DISCHARGE_ATR -> DOO_CHARGE_VENT : [after(VENT_WIDTH, msec)]
  DOO_DISCHARGE_VENT -> DOO_CHARGE_ATR : [after(ATR_WIDTH, msec)]
  VOO_CHARGE -> VOO_DISCHARGE [order 1] : after(BEAT_PERIOD - VENT_WIDTH, msec)
  IDLE -> VOO_CHARGE [order 1] : [(PACE_MODE == 1) || (PACE_MODE == 5)]
  VOO_DISCHARGE -> VOO_CHARGE : after(VENT_WIDTH, msec)
  IDLE -> IDLE [order 6] : [(PACE_MODE == 0) && (after(50,msec))]
  (default) -> IDLE
  DOO_CHARGE_VENT -> DOO_DISCHARGE_VENT : [after(AV_DELAY, msec)]
  IDLE -> VVI_CHARGE [order 4] : [(PACE_MODE == 3) || (PACE_MODE == 7)]
  IDLE -> AAI_CHARGE [order 5] : [(PACE_MODE == 4) || (PACE_MODE == 8)]
  IDLE -> DDD_CHARGE_ATR [order 3] : [(PACE_MODE == 11) || (PACE_MODE == 12)]
  DDD_CHARGE_ATR -> IDLE [order 1] : [(PACE_MODE ~= 11) && (PACE_MODE ~= 12)]
  AAI_CHARGE -> IDLE [order 3] : [(PACE_MODE ~= 4) && (PACE_MODE ~= 8)]
  VVI_CHARGE -> IDLE [order 3] : [(PACE_MODE ~= 3) && (PACE_MODE ~= 7)]
  VVI_CHARGE -> VVI_DISCHARGE [order 1] : after(BEAT_PERIOD - VENT_WIDTH, msec)
  VVI_DISCHARGE -> VVI_CHARGE : after(VENT_WIDTH, msec)
  VVI_CHARGE -> VVI_CHARGE [order 2] : [VENT_PACE == 1]
  AAI_DISCHARGE -> AAI_CHARGE : after(ATR_WIDTH, msec)
  AAI_CHARGE -> AAI_DISCHARGE [order 1] : after(BEAT_PERIOD - ATR_WIDTH, msec)
  DDD_CHARGE_ATR -> DDD_DISCHARGE_ATR [order 2] : [after(BEAT_PERIOD - AV_DELAY - VENT_WIDTH - ATR_WIDTH, msec)]
  DDD_CHARGE_ATR -> DDD_CHARGE_VENT [order 3] : [ATR_PACE == 1]
  AAI_CHARGE -> AAI_CHARGE [order 2] : [ATR_PACE == 1]
  DDD_DISCHARGE_ATR -> DDD_CHARGE_VENT : [after(ATR_WIDTH, msec)]
  DDD_CHARGE_VENT -> DDD_CHARGE_ATR [order 1] : [VENT_PACE == 1]
  DDD_DISCHARGE_VENT -> DDD_CHARGE_ATR : [after(VENT_WIDTH, msec)]
  DDD_CHARGE_VENT -> DDD_DISCHARGE_VENT [order 2] : [after(AV_DELAY, msec)]
  data: PACE_MODE input; ATR_WIDTH input; VENT_WIDTH input; BEAT_PERIOD input; PACE_CHARGE_CTRL output; Z_ATR_CTRL output; Z_VENT_CTRL output; ATR_PACE_CTRL output; VENT_PACE_CTRL output; PACE_GND_CTRL output; ATR_GND_CTRL output; VENT_GND_CTRL output; FRONTEND_CTRL output; VENT_PACE input boolean; ATR_PACE input boolean; AV_DELAY input; VENT_RDY output uint8; ATR_RDY output uint8

== stateflow chart Assingment3_3K04_Part1/PACE_SENSING/Hold Value ==
  settings: sampleTime=0.001
  state NO_DETECT
    entry:
    OUT_PACE = false;
  state OUT_ONE
    entry:
    OUT_PACE = true;
  note: After detection, hold the detect for ten msec
      | then set it low for enough time to debounce the pace
  state HIGH_RATE
    entry:
    OUT_PACE = false;
  (default) -> NO_DETECT
  HIGH_RATE -> NO_DETECT : [after(VENT_REFRAC, msec)]
  NO_DETECT -> OUT_ONE : [PACE_DETECT == 1]
  OUT_ONE -> HIGH_RATE : [after(10, msec)]
  data: VENT_REFRAC input; PACE_DETECT input; OUT_PACE output boolean

== stateflow chart Assingment3_3K04_Part1/PACE_SENSING/Hold Value1 ==
  settings: sampleTime=0.001
  state OUT_ONE
    entry:
    OUT_PACE = true;
  state HIGH_RATE
    entry:
    OUT_PACE = false;
  state NO_DETECT
    entry:
    OUT_PACE = false;
  note: After detection, hold the detect for ten msec
      | then set it low for enough time to debounce the pace
  HIGH_RATE -> NO_DETECT : [after(ATR_REFRAC, msec)]
  (default) -> NO_DETECT
  NO_DETECT -> OUT_ONE : [PACE_DETECT == 1]
  OUT_ONE -> HIGH_RATE : [after(10, msec)]
  data: ATR_REFRAC input; PACE_DETECT input; OUT_PACE output boolean
